simulink model "CCVS_lin_in_comm_out_diff"  (Simulink 7.5)
settings: Solver=ode45  StartTime=0.0  StopTime=10.0  RelTol=1e-3
settings Model: Creator=tugui_cat  LastModifiedBy=tugui
settings DebuggingCC: StrictBusMsg=Warning

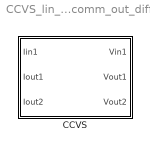
== system CCVS_lin_in_comm_out_diff ==
  CCVS : Subsystem  mask{Num_TF_dir1=1, Den_TF_dir1=1, Num_Zin1=1, Den_Zin1=1, Num_TF_inv1=1, Den_TF_inv1=1, Num_Zout1=1, Den_Zout1=1, Num_TF_dir2=1, Den_TF_dir2=1, Num_TF_inv2=1, Den_TF_inv2=1, Num_Zout2=1, Den_Zout2=1, Num_Zout_diff1=1, Den_Zout_diff1=1, Num_Zout_diff2=1, Den_Zout_diff2=1, OffIn11=0, OffIn12=0, OffOut11=0, OffOut12=0, OffOut21=0, OffOut22=0}

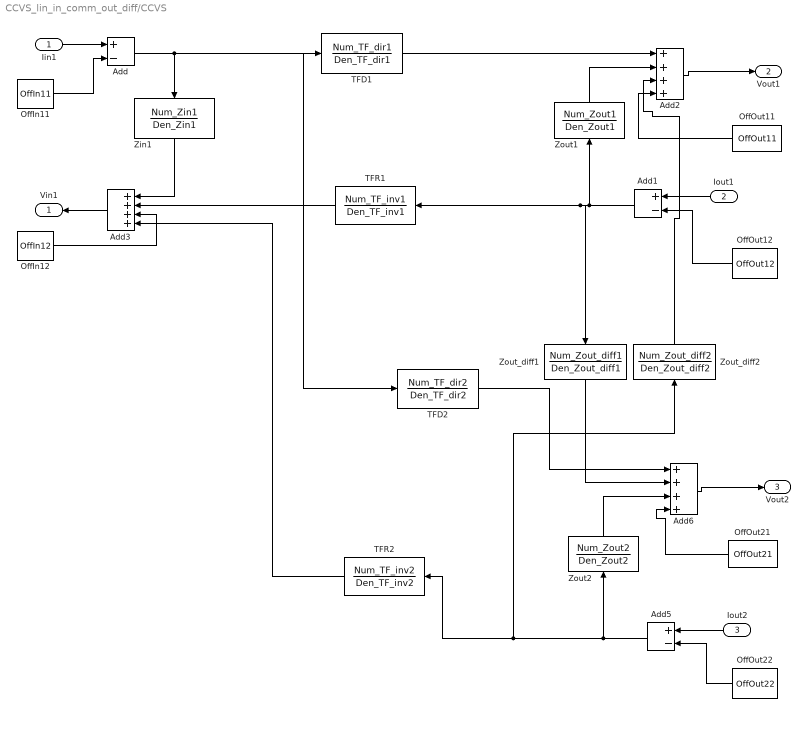
== system CCVS_lin_in_comm_out_diff/CCVS ==
  Iin1 : Inport
  Iout1 : Inport  Port=2
  Iout2 : Inport  Port=3
  Add : Sum  Inputs=+-  OutDataType=fixdt(1, 16)  OutScaling=2^-10
  Add1 : Sum  Inputs=+-  OutDataType=fixdt(1, 16)  OutScaling=2^-10
  Add2 : Sum  Inputs=++++  OutDataType=fixdt(1, 16)  OutScaling=2^-10
  Add3 : Sum  Inputs=++++  OutDataType=fixdt(1, 16)  OutScaling=2^-10
  Add5 : Sum  Inputs=+-  OutDataType=fixdt(1, 16)  OutScaling=2^-10
  Add6 : Sum  Inputs=++++  OutDataType=fixdt(1, 16)  OutScaling=2^-10
  OffIn11 : Constant  Value=OffIn11  OutDataType=fixdt(1, 16)  OutScaling=2^0
  OffIn12 : Constant  Value=OffIn12  OutDataType=fixdt(1, 16)  OutScaling=2^0
  OffOut11 : Constant  Value=OffOut11  OutDataType=fixdt(1, 16)  OutScaling=2^0
  OffOut12 : Constant  Value=OffOut12  OutDataType=fixdt(1, 16)  OutScaling=2^0
  OffOut21 : Constant  Value=OffOut21  OutDataType=fixdt(1, 16)  OutScaling=2^0
  OffOut22 : Constant  Value=OffOut22  OutDataType=fixdt(1, 16)  OutScaling=2^0
  TFD1 : TransferFcn  Numerator=Num_TF_dir1  Denominator=Den_TF_dir1
  TFD2 : TransferFcn  Numerator=Num_TF_dir2  Denominator=Den_TF_dir2
  TFR1 : TransferFcn  Numerator=Num_TF_inv1  Denominator=Den_TF_inv1
  TFR2 : TransferFcn  Numerator=Num_TF_inv2  Denominator=Den_TF_inv2
  Zin1 : TransferFcn  Numerator=Num_Zin1  Denominator=Den_Zin1
  Zout1 : TransferFcn  Numerator=Num_Zout1  Denominator=Den_Zout1
  Zout2 : TransferFcn  Numerator=Num_Zout2  Denominator=Den_Zout2
  Zout_diff1 : TransferFcn  Numerator=Num_Zout_diff1  Denominator=Den_Zout_diff1
  Zout_diff2 : TransferFcn  Numerator=Num_Zout_diff2  Denominator=Den_Zout_diff2
  Vin1 : Outport
  Vout1 : Outport  Port=2
  Vout2 : Outport  Port=3
  wires:
  TFD1/1 -> Add2/1
  Add3/1 -> Vin1/1
  Zin1/1 -> Add3/1
  TFR1/1 -> Add3/2
  Zout1/1 -> Add2/2
  Iin1/1 -> Add/1
  Add/1 -> Zin1/1, TFD1/1, TFD2/1
  OffIn11/1 -> Add/2
  Iout1/1 -> Add1/1
  Add1/1 -> Zout1/1, Zout_diff1/1, TFR1/1
  OffOut12/1 -> Add1/2
  TFR2/1 -> Add3/4
  Iout2/1 -> Add5/1
  Add5/1 -> Zout2/1, Zout_diff2/1, TFR2/1
  OffOut22/1 -> Add5/2
  Zout2/1 -> Add6/3
  TFD2/1 -> Add6/1
  OffIn12/1 -> Add3/3
  OffOut21/1 -> Add6/4
  OffOut11/1 -> Add2/4
  Add2/1 -> Vout1/1
  Add6/1 -> Vout2/1
  Zout_diff1/1 -> Add6/2
  Zout_diff2/1 -> Add2/3
